simulink model "MPC_6wd6ws"  (R2023a)
settings: Solver=VariableStepAuto  StartTime=0.0  StopTime=10.0  RelTol=1e-3
libraries: mpclib x1
settings Model: Creator=NGOC MAI  LastModifiedBy=NGOC MAI

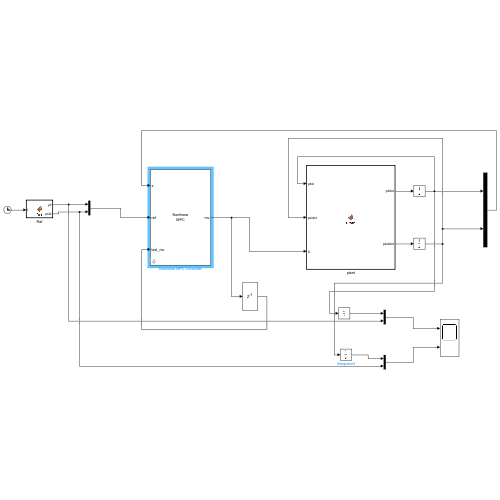
[thumbnail: Simulink's stored preview of the top-level diagram]
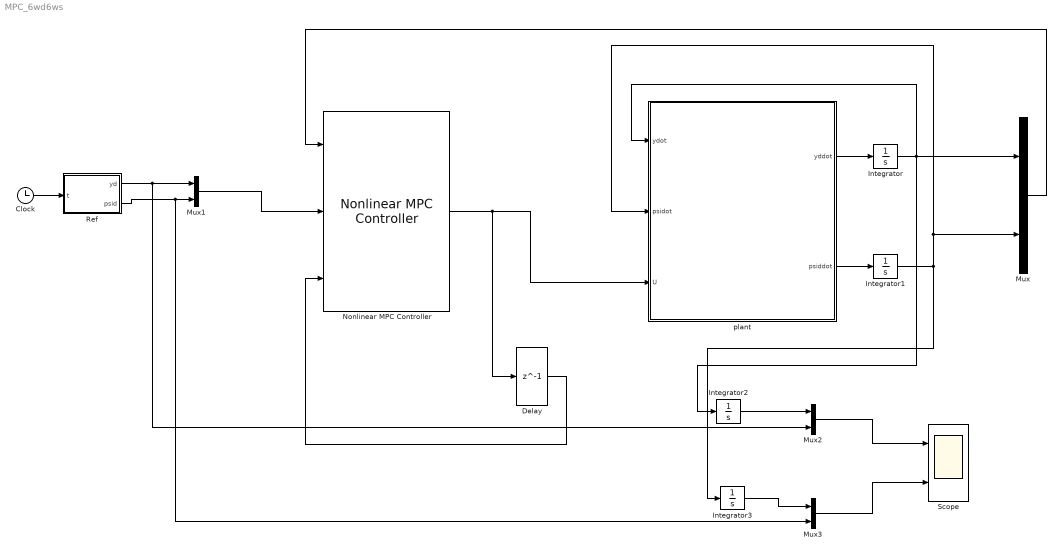
== system MPC_6wd6ws ==
  Clock : Clock
  Delay : Delay  DelayLength=1  InitialCondition=0
  Integrator{,1..3} (4 alike) : Integrator
  Mux{,1..3} (4 alike) : Mux  Inputs=2
  Nonlinear MPC Controller : mpclib/Nonlinear MPC Controller  nlmpcobj=nlobj  UseObjectTs=on  UseMEX=off  md_enabled=off  mvtarget_enabled=off  param_enabled=off  cost_enabled=off  mvseq_enabled=off  stateseq_enabled=off  ovseq_enabled=off  slack_enabled=off  status_enabled=off  ov_min=off  ov_max=off  mv_min=off  mv_max=off  mvrate_min=off  mvrate_max=off  state_min=off  state_max=off  ov_weight=off  mv_weight=off  mvrate_weight=off  ecr_weight=off  nlp_initialize=off
  Ref : MATLAB Function  TreatAsAtomicUnit=on
  Scope : Scope  NumInputPorts=2
  plant : MATLAB Function  TreatAsAtomicUnit=on
  wires:
  plant/1(yddot) -> Integrator/1
  Integrator/1 -> plant/1(ydot), Integrator2/1, Mux/1
  plant/2(psiddot) -> Integrator1/1
  Integrator1/1 -> Integrator3/1, Mux/2, plant/2(psidot)
  Nonlinear MPC Controller/1 -> Delay/1, plant/3(U)
  Delay/1 -> Nonlinear MPC Controller/3
  Mux/1 -> Nonlinear MPC Controller/1
  Clock/1 -> Ref/1(t)
  Ref/1(yd) -> Mux2/2, Mux1/1
  Ref/2(psid) -> Mux3/2, Mux1/2
  Mux1/1 -> Nonlinear MPC Controller/2
  Integrator2/1 -> Mux2/1
  Integrator3/1 -> Mux3/1
  Mux2/1 -> Scope/1
  Mux3/1 -> Scope/2

== matlab function MPC_6wd6ws/Ref ==
  data: t input; yd output; psid output
function [yd,psid]= fcn(t)
%yd=10*(tanh(3*t-35)-tanh(3*t-6));
%psid=(sech(3*t-60))^2-(sech(3*t-35)^2);
yd = 1.5*(tanh(t-6) - tanh(t-14));
psid = 1.5*(-(sech(t-14))^2 + (sech(t-6))^2)/20;
end

== matlab function MPC_6wd6ws/plant ==
  data: ydot input; yddot output; psidot input; U input; psiddot output
function [yddot, psiddot] = State(ydot, psidot, U)
m=1350; %kg
J=1350; %kgm^2
cf=55000; %N/rad
cm=100000; %N/rad
cr=120000; %N/rad
lf=2.5; %m
lm=0.5; %m
lr=3; %m
vx=20; %m/s
a1 = (-2*lf*cf - 2*lm*cm + 2*lr*cr)/(J*vx);
a2 = 2*((lf^2)*cf + (lm^2)*cm - (lr^2)*cr)/(J*vx);
a3 = 2*lf*cf/J;
a4 = 2*lm*cm/J;
a5 = -2*lr*cr/J;

b1 = 2*(-cf - cr - cm)/(m*vx);
b2 = 2*(lf*cf + lm*cm + lr*cr)/(m*vx)-vx;
b3 = 2*cf/m;
b4 = 2*cm/m;
b5 = 2*cr/m;

X = [ydot ; psidot];

A = [b1 , b2 ; a1 , a2];
B = [b3 , b4 , b5 ; a3 , a4 , a5];
Xdot = A*X + B*U;

yddot = Xdot(1);
psiddot = Xdot(2);
end
